simulink model "dsm_3rd_order_ct_10mhz_topology_model"  (R2025b)
settings: Solver=ode4  StartTime=0.0  StopTime=0.0008191  FixedStep=3.125e-09  RelTol=1e-3
model workspace (MAT data in the model file):
  Ac_ct = [0  0  0; 1  0  -0.00578297132876; 0  1  0]
  Bc_ct = [1  -1; 0  0; 0  0]
  Cc_ct = [1.5500645211 1.41393998955 0.600426824781]
  Dc_ct = [0 0]
  Ts_dsm = 1e-07
  x0_ct = [0; 0; 0]
undefined symbols (not defined in the file or in its folder): dsm_quantizer
settings Model: Creator=sli767  LastModifiedBy=sli767

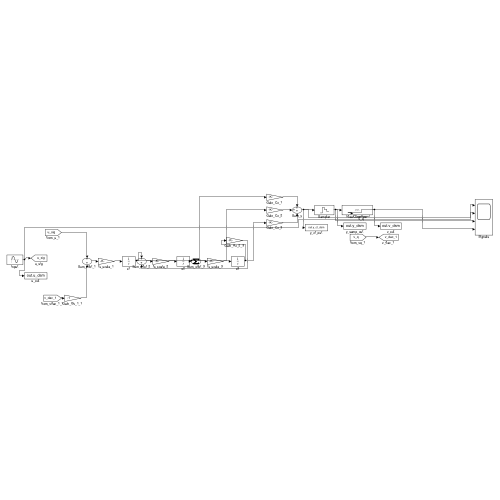
[thumbnail: Simulink's stored preview of the top-level diagram]
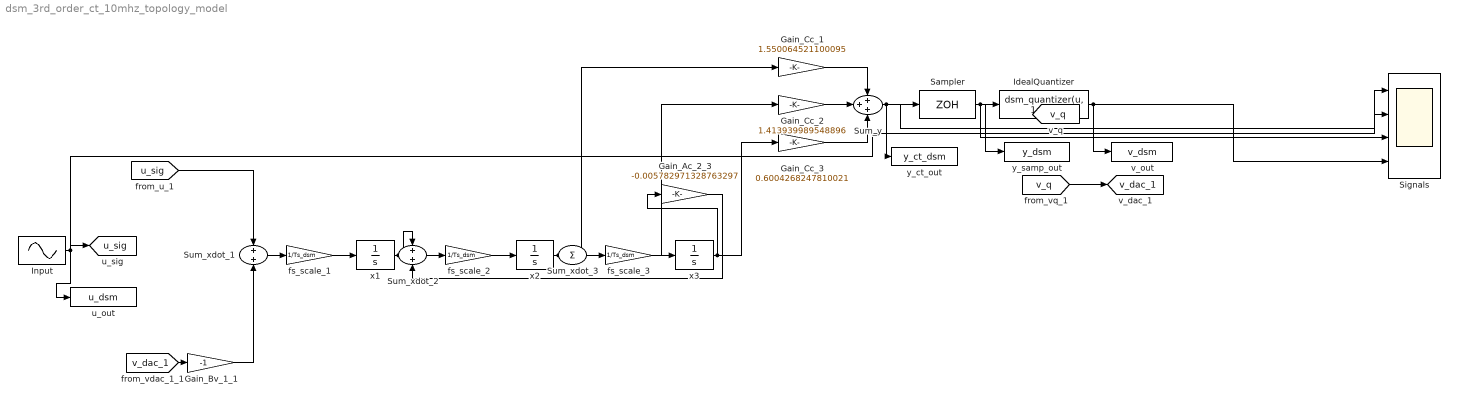
== system dsm_3rd_order_ct_10mhz_topology_model ==
  Gain_Ac_2_3 : Gain  Gain=-0.005782971328763297
  Gain_Bv_1_1 : Gain  Gain=-1
  Gain_Cc_1 : Gain  Gain=1.550064521100095
  Gain_Cc_2 : Gain  Gain=1.413939989548896
  Gain_Cc_3 : Gain  Gain=0.6004268247810021
  IdealQuantizer : MATLABFcn  MATLABFcn=dsm_quantizer(u, 1, 16)
  Input : Sin  Amplitude=0.5  Frequency=368155.3890925539  SampleTime=0
  Sampler : ZeroOrderHold  SampleTime=Ts_dsm
  Signals : Scope  NumInputPorts=4
  Sum_xdot_1 : Sum
  Sum_xdot_2 : Sum
  Sum_xdot_3 : Sum  Inputs=+
  Sum_y : Sum  Inputs=+++
  fs_scale_1 : Gain  Gain=1/Ts_dsm
  fs_scale_2 : Gain  Gain=1/Ts_dsm
  fs_scale_3 : Gain  Gain=1/Ts_dsm
  u_out : ToWorkspace  VariableName=u_dsm  SampleTime=-1
  v_out : ToWorkspace  VariableName=v_dsm  SampleTime=-1
  x1 : Integrator  InitialCondition=x0_ct(1)
  x2 : Integrator  InitialCondition=x0_ct(2)
  x3 : Integrator  InitialCondition=x0_ct(3)
  y_ct_out : ToWorkspace  VariableName=y_ct_dsm  SampleTime=-1
  y_samp_out : ToWorkspace  VariableName=y_dsm  SampleTime=-1
  tag scope: u_sig=global, v_dac_1=global, v_q=global
  wires:
  Input/1 -> [u_sig], u_out/1, Signals/1
  [v_q] -> [v_dac_1]
  Sum_xdot_1/1 -> fs_scale_1/1
  fs_scale_1/1 -> x1/1
  Sum_xdot_2/1 -> fs_scale_2/1
  fs_scale_2/1 -> x2/1
  Sum_xdot_3/1 -> fs_scale_3/1
  fs_scale_3/1 -> x3/1
  [u_sig] -> Sum_xdot_1/1
  [v_dac_1] -> Gain_Bv_1_1/1
  Gain_Bv_1_1/1 -> Sum_xdot_1/2
  x1/1 -> Sum_xdot_2/1, Gain_Cc_1/1
  x3/1 -> Gain_Ac_2_3/1, Gain_Cc_3/1
  Gain_Ac_2_3/1 -> Sum_xdot_2/2
  x2/1 -> Sum_xdot_3/1, Gain_Cc_2/1
  Gain_Cc_1/1 -> Sum_y/1
  Gain_Cc_2/1 -> Sum_y/2
  Gain_Cc_3/1 -> Sum_y/3
  Sum_y/1 -> Sampler/1, y_ct_out/1, Signals/2
  Sampler/1 -> IdealQuantizer/1, y_samp_out/1, Signals/3
  IdealQuantizer/1 -> [v_q], v_out/1, Signals/4
